simulink model "helicoptertemplate_mpc_offset_2"  (R2021b)
settings: Solver=ode45  StartTime=0.0  StopTime=Tsim  RelTol=1e-3
InitFcn:
  | hwinit
values from neighbouring files (symbols this model uses):
  A = sysd.A    [MPC_Reference_track.m]    (also in MPC_Reference_track_offset.m; MPC_init_v2.m; MPC_init_v3.m; modelDynamics.m = [0, 1; -(1/J)*g*Mcw*L1*cos(-0.38), -(1/J)*C_alpha])
  B = sysd.B    [MPC_Reference_track.m]    (also in MPC_Reference_track_offset.m; MPC_init_v2.m; MPC_init_v3.m; modelDynamics.m = [0; (1/J)*L2])
  C = sysd.C    [MPC_Reference_track.m]    (also in MPC_Reference_track_offset.m; MPC_init_v2.m; MPC_init_v3.m; modelDynamics.m = [1, 0])
  H = S'*Qbar*S + Rbar    [costgen.m]    (also in costgen_delta.m = S' * Qbar * S + Delta' * Rbar * Delta)
  h = 0.01    [MPC_Reference_track.m]    (also in MPC_Reference_track_offset.m; MPC_init_v2.m; MPC_init_v3.m; costgen.m = [hx0 hxref huref])
  sysd = c2d(sys, h)    [MPC_Reference_track.m]    (also in MPC_Reference_track_offset.m; MPC_init_v2.m; MPC_init_v3.m)
  y_ref = -[0.2*ones(1,T_steps/4), 0.3*ones(1,T_steps/4), 0.1*ones(1,T_steps/4), 0.38*ones(1,(T_steps/4)+1),]'    [MPC_Reference_track.m]    (also in MPC_Reference_track_offset.m; MPC_init_v2.m = -0.2; MPC_init_v3.m = -0.1)
undefined symbols (not defined in the file or in its folder): adingain, adinoffs, DiscIntNeverNeededParam, Discrete, h_cost, HeliMexHandle, Time
libraries: ctrlSharedLib x2
settings Model: Creator=fkzhang  LastModifiedBy=rjvanderhorst
settings SolverCC: AlgebraicLoopSolver=TrustRegion
settings DataIOCC: LimitDataPoints=on  SaveFormat=Array  ReturnWorkspaceOutputs=off
settings OptimizationCC: BlockReduction=off  BooleanDataType=off  LifeSpan=inf
settings DebuggingCC: SaveWithParameterizedLinksMsg=none  UnderspecifiedInitializationDetection=Classic  MergeDetectMultiDrivingBlocksExec=none  SignalResolutionControl=TryResolveAllWithWarning  AllowSymbolicDim=off  SFUnexpectedBacktrackingDiag=warning  SFNoUnconditionalDefaultTransitionDiag=warning  SFExecutionAtInitializationDiag=none  SFMachineParentedDataDiag=warning  ArithmeticOperatorsInVariantConditions=warning
settings HardwareCC: ProdBitPerPointer=32  ProdBitPerSizeT=32  ProdBitPerPtrDiffT=32  ProdLargestAtomicFloat=None  ProdIntDivRoundTo=Undefined  ProdEndianess=Unspecified  ProdWordSize=32  ProdHWDeviceType=32-bit Generic  TargetUnknown=on
settings ModelReferenceCC: PropagateSignalLabelsOutOfModel=off
settings SFSimCC: SimUseLocalCustomCode=off  CustomCodeUndefinedFunction=UseInterfaceOnly
settings RTWCC: RTWUseLocalCustomCode=off
settings CodeAppCC: StateflowObjectComments=on
settings GRTTargetCC: TargetLangStandard=C89/C90 (ANSI)
settings ConfigComp: CovMetricSettings=dw  CovSaveCumulativeToWorkspaceVar=on  CovSaveSingleToWorkspaceVar=on  CovExternalEMLEnable=off  CovSFcnEnable=off

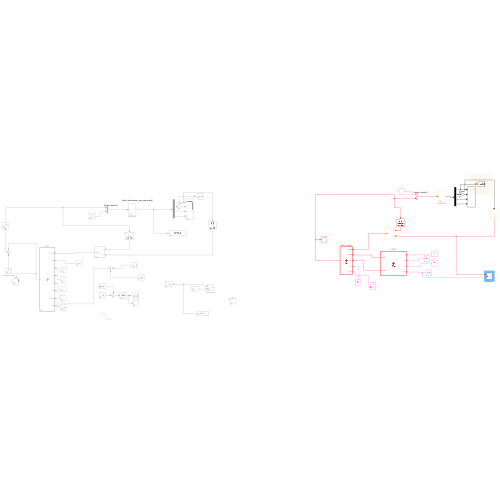
[thumbnail: Simulink's stored preview of the top-level diagram]
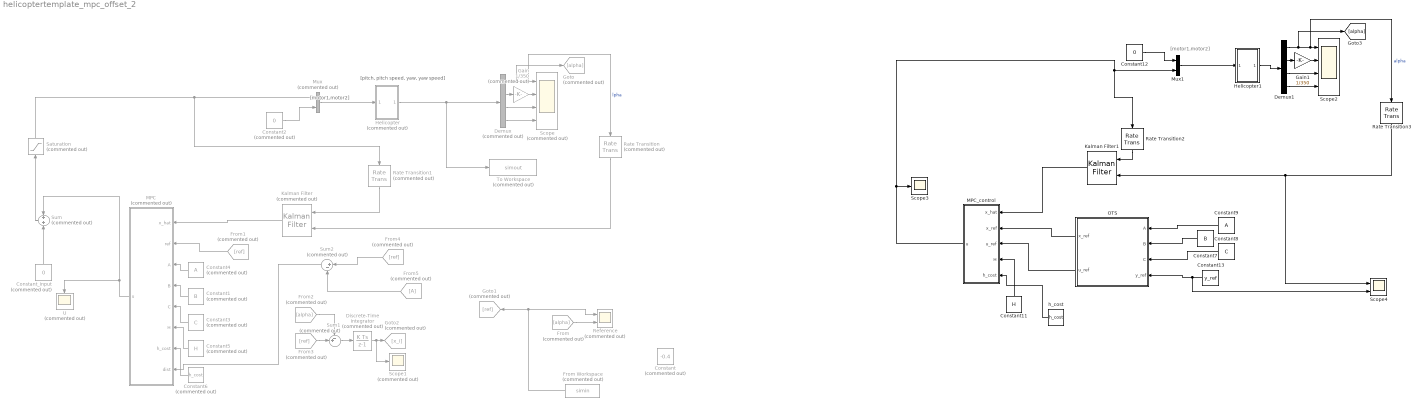
== system helicoptertemplate_mpc_offset_2 ==
  note: [pitch, pitch speed, yaw, yaw speed]
  note: [motor1,motor2]
  note: [motor1,motor2]
  Constant : Constant  Commented=on  Value=-0.4
  Constant1 : Constant  Commented=on  Value=B  VectorParams1D=off
  Constant11 : Constant  Value=H
  Constant12 : Constant  Value=0
  Constant13 : Constant  Value=y_ref
  Constant2 : Constant  Commented=on  Value=0
  Constant3 : Constant  Commented=on  Value=C  VectorParams1D=off
  Constant4 : Constant  Commented=on  Value=A
  Constant5 : Constant  Commented=on  Value=H
  Constant6 : Constant  Commented=on  Value=h_cost
  Constant7 : Constant  Value=B  VectorParams1D=off
  Constant8 : Constant  Value=C  VectorParams1D=off
  Constant9 : Constant  Value=A
  Constant_input : Constant  Commented=on  Value=0
  Demux : Demux  Commented=on
  Demux1 : Demux
  Discrete-Time Integrator : DiscreteIntegrator  Commented=on  SampleTime=-1  ICPrevOutput=DiscIntNeverNeededParam  ICPrevScaledInput=DiscIntNeverNeededParam
  From : From  Commented=on  GotoTag=alpha
  From Workspace : FromWorkspace  Commented=on  VariableName=simin
  From1 : From  Commented=on  GotoTag=ref
  From2 : From  Commented=on  GotoTag=alpha
  From3 : From  Commented=on  GotoTag=ref
  From4 : From  Commented=on  GotoTag=ref
  From5 : From  Commented=on
  Gain : Gain  Commented=on  Gain=1/350
  Gain1 : Gain  Gain=1/350
  Goto : Goto  Commented=on  GotoTag=alpha
  Goto1 : Goto  Commented=on  GotoTag=ref
  Goto2 : Goto  Commented=on  GotoTag=x_i
  Helicopter : Subsystem  Commented=on  mask{Ts=h}
      mask prompts: Ts "sampletime"
      mask init:
      | sf_heli_init
      mask Display:
      | port_label('input',1,'u');
      | port_label('output',1,'y');
  Helicopter1 : Subsystem  mask{Ts=h}
      mask prompts: Ts "sampletime"
      mask init:
      | sf_heli_init
      mask Display:
      | port_label('input',1,'u');
      | port_label('output',1,'y');
  Kalman Filter : ctrlSharedLib/Kalman Filter  Commented=on  TimeDomain=Discrete-Time  UseCurrentEstimator=on  ModelSource=Individual A, B, C, D matrices  ModelSourceVariable=ss(0.95,1,1,0,1)  A=A  B=B  C=C  D=sysd.D  NumberOfStates=1  NumberOfInputs=1  NumberOfOutputs=1  InitialEstimateSource=Dialog  X0=[0; 0]  P0=10  UseK=off  UseGH=off  NumberOfProcessNoiseInputs=1  G=1  TimeInvariantG=on  H=0  TimeInvariantH=on  Q=0.05  TimeInvariantQ=on  R=1  TimeInvariantR=on  N=0  TimeInvariantN=on  AddInputPort=on  AddEnablePort=off  OutputEstimatedY=off  OutputP=off  Ts=h
  Kalman Filter1 : ctrlSharedLib/Kalman Filter  TimeDomain=Discrete-Time  UseCurrentEstimator=on  ModelSource=Individual A, B, C, D matrices  ModelSourceVariable=ss(0.95,1,1,0,1)  A=sysd.A  B=sysd.B  C=sysd.C  D=0  NumberOfStates=1  NumberOfInputs=1  NumberOfOutputs=1  InitialEstimateSource=Dialog  X0=[0;0]  P0=10  UseK=off  UseGH=off  NumberOfProcessNoiseInputs=1  G=1  TimeInvariantG=on  H=0  TimeInvariantH=on  Q=0.05  TimeInvariantQ=on  R=1  TimeInvariantR=on  N=0  TimeInvariantN=on  AddInputPort=on  AddEnablePort=off  OutputEstimatedY=off  OutputP=off  Ts=h
  MPC : MATLAB Function  Commented=on  TreatAsAtomicUnit=on
  MPC_control : MATLAB Function  TreatAsAtomicUnit=on
  Mux : Mux  Commented=on  Inputs=2
  Mux1 : Mux  Inputs=2
  OTS : MATLAB Function  TreatAsAtomicUnit=on
  Rate Transition : RateTransition  Commented=on  OutPortSampleTime=h
  Rate Transition1 : RateTransition  Commented=on  OutPortSampleTime=h
  Rate Transition2 : RateTransition  OutPortSampleTime=h
  Rate Transition3 : RateTransition  OutPortSampleTime=h
  Reference : Scope  Commented=on  NumInputPorts=2
  Saturation : Saturate  Commented=on  UpperLimit=1  LowerLimit=-1
  Scope : Scope  Commented=on  NumInputPorts=4
  Scope1 : Scope  Commented=on
  Scope2 : Scope  NumInputPorts=4
  Scope3 : Scope
  Scope4 : Scope  NumInputPorts=2
  Sum : Sum  Commented=on
  Sum1 : Sum  Commented=on  Inputs=-+|
  Sum2 : Sum  Commented=on  Inputs=|+-
  To Workspace : ToWorkspace  Commented=on  VariableName=simout  SaveFormat=Structure With Time  SampleTime=-1
  U : Scope  Commented=on
  h_cost : Constant  Value=h_cost
  wires:
  Helicopter/1(Out1) -> To Workspace/1, Demux/1
  Mux/1 -> Helicopter/1(In1)
  Constant2/1 -> Mux/2
  Demux/3 -> Scope/3
  Demux/4 -> Scope/4
  Demux/2 -> Gain/1
  Gain/1 -> Scope/2
  Demux/1 -> Goto/1, Rate Transition/1, Scope/1  "lpha"
  Constant_input/1 -> Sum/2
  Sum/1 -> Saturation/1
  MPC/1(u) -> Sum/1, U/1
  Saturation/1 -> Rate Transition1/1, Mux/1
  Rate Transition/1 -> Kalman Filter/2
  From/1 -> Reference/2
  From Workspace/1 -> Reference/1, Goto1/1
  From2/1 -> Sum1/1
  From3/1 -> Sum1/2
  Sum1/1 -> Discrete-Time Integrator/1
  Discrete-Time Integrator/1 -> Scope1/1, Goto2/1
  Constant1/1 -> MPC/4(B)
  Constant3/1 -> MPC/5(C)
  Constant4/1 -> MPC/3(A)
  Constant5/1 -> MPC/6(H)
  Constant6/1 -> MPC/7(h_cost)
  Rate Transition1/1 -> Kalman Filter/1
  Sum2/1 -> MPC/8(dist)
  From5/1 -> Sum2/2
  From4/1 -> Sum2/1
  Kalman Filter/1 -> MPC/1(x_hat)
  From1/1 -> MPC/2(ref)
  ? -> ?
  Constant9/1 -> OTS/1(A)
  Constant8/1 -> OTS/3(C)
  Constant7/1 -> OTS/2(B)
  Constant13/1 -> Scope4/2, OTS/4(y_ref)
  OTS/1(x_ref) -> MPC_control/2(x_ref)
  OTS/2(u_ref) -> MPC_control/3(u_ref)
  Constant11/1 -> MPC_control/4(H)
  h_cost/1 -> MPC_control/5(h_cost)
  Constant12/1 -> Mux1/1
  Mux1/1 -> Helicopter1/1(In1)
  Rate Transition2/1 -> Kalman Filter1/1
  MPC_control/1(u) -> Mux1/2, Rate Transition2/1, Scope3/1
  Demux1/3 -> Scope2/3
  Demux1/1 -> [alpha], Rate Transition3/1, Scope2/1  "alpha"
  Helicopter1/1(Out1) -> Demux1/1
  Demux1/4 -> Scope2/4
  Demux1/2 -> Gain1/1
  Gain1/1 -> Scope2/2
  Rate Transition3/1 -> Scope4/1, Kalman Filter1/2
  Kalman Filter1/1 -> MPC_control/1(x_hat)

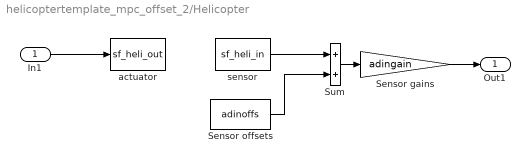
== system helicoptertemplate_mpc_offset_2/Helicopter ==
  In1 : Inport
  Sensor gains : Gain  Gain=adingain
  Sensor offsets : Constant  Value=adinoffs
  Sum : Sum
  actuator : M-S-Function  FunctionName=sf_heli_out  Parameters=HeliMexHandle,Ts
  sensor : M-S-Function  FunctionName=sf_heli_in  Parameters=HeliMexHandle
  Out1 : Outport
  wires:
  sensor/1 -> Sum/1
  In1/1 -> actuator/1
  Sensor offsets/1 -> Sum/2
  Sum/1 -> Sensor gains/1
  Sensor gains/1 -> Out1/1

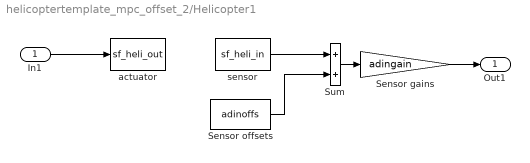
== system helicoptertemplate_mpc_offset_2/Helicopter1 ==
  In1 : Inport
  Sensor gains : Gain  Gain=adingain
  Sensor offsets : Constant  Value=adinoffs
  Sum : Sum
  actuator : M-S-Function  FunctionName=sf_heli_out  Parameters=HeliMexHandle,Ts
  sensor : M-S-Function  FunctionName=sf_heli_in  Parameters=HeliMexHandle
  Out1 : Outport
  wires:
  sensor/1 -> Sum/1
  In1/1 -> actuator/1
  Sensor offsets/1 -> Sum/2
  Sum/1 -> Sensor gains/1
  Sensor gains/1 -> Out1/1

== matlab function helicoptertemplate_mpc_offset_2/MPC_control ==
  data: x_hat input; u output; x_ref input; u_ref input; H input; h_cost input
function u = fcn(x_hat, x_ref, u_ref, H, h_cost)
    u = 0;
    coder.extrinsic('quadprog');
    coder.extrinsic('warning');

    x_0=x_hat;
    N = 10;
    lb = -1*ones(N,1);
    ub = -1*lb;
    options = optimset('Display', 'off');
    warning('off', 'all');
    uN = quadprog(H,(h_cost*[x_0; x_ref; u_ref]),[],[],[],[],lb,ub,[],options);
    % Select the first input only
    warning('on', 'all');
    u = uN(1);

== matlab function helicoptertemplate_mpc_offset_2/MPC ==
  data: x_hat input; ref input; A input; B input; u output; C input; H input; h_cost input; dist input
function u = fcn(x_hat, ref , A, B, C, H, h_cost, dist)
      
    u = zeros(1,1); % Define the output type for the extrinsic call.
    
    N = 20; %prediction horizon
    coder.extrinsic('quadprog');
%     A_OT = [eye(2)-A, -B; C, zeros(1,1)];
%     disp(size(A_OT))
%     B_OT = [zeros(2,1); ref];
%     
%     H_ots = [0 0 0;
%              0 0 0;
%              0 0 1];
%     
%     lb_ots = [-10000; 0; -1];
%     ub_ots = -lb_ots;
%     
%     %options = optimoptions('fmincon', 'Algorithm','sqp');
%     OTS = quadprog(H_ots,[],[],[],A_OT,B_OT,lb_ots,ub_ots,[]);
%     x_ref = OTS(1:2);
%     u_ref = OTS(3);

    x_ref = [ref;0];
    u_ref = ref/0.6599;
    %%%%%%%%%%%%%%%%%%%%%%%%%%%OTS%%%%%%%%%%%%%%%%%%%%%%%%%%%%


    

    %%%%%%%%%%%%%%%%%%%%%%%%%%%MPC%%%%%%%%%%%%%%%%%%%%%%%%%%%%
    x_0=x_hat(1:2);
    
    lb = -1*ones(N,1);
    ub = -1*lb;
    uN = quadprog(H,(h_cost*[x_0; x_ref; u_ref]),[],[],[],[],lb,ub,[]);

    % Select the first input only
    u=uN(1);
    u = -1*u;
end

== matlab function helicoptertemplate_mpc_offset_2/OTS ==
  data: A input; x_ref output; B input; C input; y_ref input; u_ref output
function [x_ref, u_ref] = fcn(A, B, C, y_ref)
    x_ref = [0; 0];
    u_ref = [0];
    coder.extrinsic('quadprog');
    coder.extrinsic('warning');

    A_OT = [eye(2)-A, -B; C, 0];
    B_OT = [zeros(2,1); y_ref];
    
    H_ots = [0 0 0;
             0 0 0;
             0 0 1];
    
    lb_ots = [-10000; 0; -1];
    ub_ots = -lb_ots;
    
    options = optimset('Display', 'on');
    OTS = quadprog(H_ots,[],[],[],A_OT,B_OT,lb_ots,ub_ots,[],options)
    x_ref = OTS(1:2);
    u_ref = OTS(3);
